simulink model "Cardiovascularmodel"  (Simulink 7.4)
settings: Solver=ode45  StartTime=0.0  StopTime=10.0  RelTol=1e-3
undefined symbols (not defined in the file): magnitude
(part 2 of 2)

== system Cardiovascularmodel/26 - 34/0.0.34i ==
  fsp : Inport  OutDataType=fixdt(1, 16)  OutScaling=2^0
  Constant : Constant  Value=0  OutDataType=fixdt(1, 16)  OutScaling=2^0
  Constant1 : Constant  OutDataType=fixdt(1, 16)  OutScaling=2^0
  D(V(u,ev)) : Constant  Value=5  OutDataType=fixdt(1, 16)  OutScaling=2^0
  G(V(e,sv)) : Constant  Value=-74.21  OutDataType=fixdt(1, 16)  OutScaling=2^0
  Math Function : Math  Operator=log  OutDataType=fixdt(1, 16)  OutScaling=2^0  SaturateOnIntegerOverflow=on
  Product : Product  OutDataType=fixdt(1, 16)  OutScaling=2^0  RndMeth=Zero
  Subtract1 : Sum  Inputs=++-  OutDataType=fixdt(1, 16)  OutScaling=2^-10
  Switch : Switch  Threshold=2.66  OutDataType=fixdt(1, 16)  OutScaling=2^0
  Variable Time Delay : VariableTransportDelay  MaximumDelay=10
  f(es,min) : Constant  Value=2.66  OutDataType=fixdt(1, 16)  OutScaling=2^0
  sigma(V(e,sv)) : Outport  OutDataType=fixdt(1, 16)  OutScaling=2^0
  wires:
  fsp/1 -> Switch/2, Variable Time Delay/1
  Switch/1 -> sigma(V(e,sv))/1
  Constant/1 -> Switch/3
  G(V(e,sv))/1 -> Product/1
  Product/1 -> Switch/1
  f(es,min)/1 -> Subtract1/3
  Variable Time Delay/1 -> Subtract1/2
  Constant1/1 -> Subtract1/1
  Subtract1/1 -> Math Function/1
  Math Function/1 -> Product/2
  D(V(u,ev))/1 -> Variable Time Delay/2

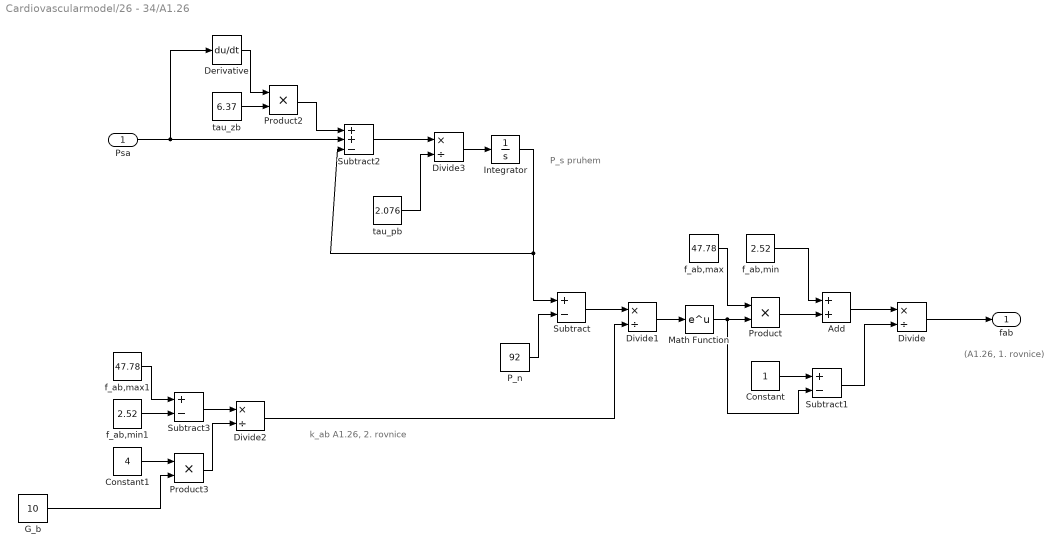
== system Cardiovascularmodel/26 - 34/A1.26 ==
  note: k_ab
      | A1.26, 2. rovnice
  note: P_s pruhem
  note: (A1.26, 1. rovnice)
  Psa : Inport  OutDataType=sfix(16)  OutScaling=2^0
  Add : Sum  OutDataType=sfix(16)  OutScaling=2^-10
  Constant : Constant  OutDataType=sfix(16)  OutScaling=2^0
  Constant1 : Constant  Value=4  OutDataType=sfix(16)  OutScaling=2^0
  Derivative : Derivative
  Divide : Product  Inputs=*/  OutDataType=sfix(16)  OutScaling=2^-10
  Divide1 : Product  Inputs=*/  OutDataType=sfix(16)  OutScaling=2^-10
  Divide2 : Product  Inputs=*/  OutDataType=sfix(16)  OutScaling=2^-10
  Divide3 : Product  Inputs=*/  OutDataType=fixdt(1, 16)  OutScaling=2^-10
  G_b : Constant  Value=10  OutDataType=sfix(16)  OutScaling=2^0
  Integrator : Integrator
  Math Function : Math  OutDataType=sfix(16)  OutScaling=2^0  SaturateOnIntegerOverflow=on
  P_n : Constant  Value=92  OutDataType=sfix(16)  OutScaling=2^0
  Product : Product  OutDataType=sfix(16)  OutScaling=2^0  RndMeth=Zero
  Product2 : Product  OutDataType=sfix(16)  OutScaling=2^0  RndMeth=Zero
  Product3 : Product  OutDataType=sfix(16)  OutScaling=2^0  RndMeth=Zero
  Subtract : Sum  Inputs=+-  OutDataType=sfix(16)  OutScaling=2^-10
  Subtract1 : Sum  Inputs=+-  OutDataType=sfix(16)  OutScaling=2^-10
  Subtract2 : Sum  Inputs=++-  OutDataType=sfix(16)  OutScaling=2^-10
  Subtract3 : Sum  Inputs=+-  OutDataType=sfix(16)  OutScaling=2^-10
  f_ab,max : Constant  Value=47.78  OutDataType=sfix(16)  OutScaling=2^0
  f_ab,max1 : Constant  Value=47.78  OutDataType=sfix(16)  OutScaling=2^0
  f_ab,min : Constant  Value=2.52  OutDataType=sfix(16)  OutScaling=2^0
  f_ab,min1 : Constant  Value=2.52  OutDataType=sfix(16)  OutScaling=2^0
  tau_pb : Constant  Value=2.076  OutDataType=sfix(16)  OutScaling=2^0
  tau_zb : Constant  Value=6.37  OutDataType=sfix(16)  OutScaling=2^0
  fab : Outport  OutDataType=sfix(16)  OutScaling=2^0
  wires:
  Divide/1 -> fab/1
  Add/1 -> Divide/1
  Product/1 -> Add/2
  f_ab,min/1 -> Add/1
  f_ab,max/1 -> Product/1
  Math Function/1 -> Product/2, Subtract1/2
  Divide1/1 -> Math Function/1
  Subtract/1 -> Divide1/1
  P_n/1 -> Subtract/2
  Subtract1/1 -> Divide/2
  Constant/1 -> Subtract1/1
  Psa/1 -> Subtract2/2, Derivative/1
  Product2/1 -> Subtract2/1
  tau_zb/1 -> Product2/2
  Divide2/1 -> Divide1/2
  Subtract3/1 -> Divide2/1
  f_ab,min1/1 -> Subtract3/2
  f_ab,max1/1 -> Subtract3/1
  Product3/1 -> Divide2/2
  Constant1/1 -> Product3/1
  G_b/1 -> Product3/2
  Derivative/1 -> Product2/1
  tau_pb/1 -> Divide3/2
  Subtract2/1 -> Divide3/1
  Divide3/1 -> Integrator/1
  Integrator/1 -> Subtract/1, Subtract2/3

== system Cardiovascularmodel/26 - 34/Elastance 0.0.32d ==
  delta Emax,lv : Inport  OutDataType=fixdt(1, 16)  OutScaling=2^0
  Emax,lv,0 : Constant  Value=2.392  OutDataType=fixdt(1, 16)  OutScaling=2^0
  Sum : Sum  Inputs=|++  OutDataType=fixdt(1, 16)  OutScaling=2^0
  E max,lv : Outport  OutDataType=fixdt(1, 16)  OutScaling=2^0
  wires:
  Sum/1 -> E max,lv/1
  Emax,lv,0/1 -> Sum/1
  delta Emax,lv/1 -> Sum/2

== system Cardiovascularmodel/26 - 34/Elastance dynamic 0.0.32b ==
  sigma (Emax,rv) : Inport  OutDataType=fixdt(1, 16)  OutScaling=2^0
  Constant : Constant  OutDataType=fixdt(1, 16)  OutScaling=2^0
  Constant1 : Constant  Value=-1  OutDataType=fixdt(1, 16)  OutScaling=2^0
  Divide : Product  Inputs=*/  OutDataType=fixdt(1, 16)  OutScaling=2^-10
  Integrator : Integrator
  Product : Product  OutDataType=fixdt(1, 16)  OutScaling=2^0  RndMeth=Zero
  Product1 : Product  OutDataType=fixdt(1, 16)  OutScaling=2^0  RndMeth=Zero
  Sum : Sum  Inputs=|++  OutDataType=fixdt(1, 16)  OutScaling=2^0
  tau(Emax,rv) : Constant  Value=8  OutDataType=fixdt(1, 16)  OutScaling=2^0
  delta  Emax,rv : Outport  OutDataType=fixdt(1, 16)  OutScaling=2^0
  wires:
  sigma (Emax,rv)/1 -> Sum/1
  Constant/1 -> Divide/1
  tau(Emax,rv)/1 -> Divide/2
  Divide/1 -> Product/1
  Constant1/1 -> Product1/2
  Product1/1 -> Sum/2
  Sum/1 -> Product/2
  Product/1 -> Integrator/1
  Integrator/1 -> delta  Emax,rv/1, Product1/1

== system Cardiovascularmodel/26 - 34/Elastance dynamic 0.0.32c ==
  delta Emax,rv : Inport  OutDataType=fixdt(1, 16)  OutScaling=2^0
  Emax,rv,0 : Constant  Value=1.412  OutDataType=fixdt(1, 16)  OutScaling=2^0
  Sum : Sum  Inputs=|++  OutDataType=fixdt(1, 16)  OutScaling=2^0
  E max,rv : Outport  OutDataType=fixdt(1, 16)  OutScaling=2^0
  wires:
  Sum/1 -> E max,rv/1
  Emax,rv,0/1 -> Sum/1
  delta Emax,rv/1 -> Sum/2

== system Cardiovascularmodel/26 - 34/Elastance dynamic 0.0.32e ==
  sigma (Emax,lv) : Inport  OutDataType=fixdt(1, 16)  OutScaling=2^0
  Constant : Constant  OutDataType=fixdt(1, 16)  OutScaling=2^0
  Constant1 : Constant  Value=-1  OutDataType=fixdt(1, 16)  OutScaling=2^0
  Divide : Product  Inputs=*/  OutDataType=fixdt(1, 16)  OutScaling=2^-10
  Integrator : Integrator
  Product : Product  OutDataType=fixdt(1, 16)  OutScaling=2^0  RndMeth=Zero
  Product1 : Product  OutDataType=fixdt(1, 16)  OutScaling=2^0  RndMeth=Zero
  Sum : Sum  Inputs=|++  OutDataType=fixdt(1, 16)  OutScaling=2^0
  tau(Emax,rv) : Constant  Value=8  OutDataType=fixdt(1, 16)  OutScaling=2^0
  delta  Emax,lv : Outport  OutDataType=fixdt(1, 16)  OutScaling=2^0
  wires:
  sigma (Emax,lv)/1 -> Sum/1
  Constant/1 -> Divide/1
  tau(Emax,rv)/1 -> Divide/2
  Divide/1 -> Product/1
  Constant1/1 -> Product1/2
  Product1/1 -> Sum/2
  Sum/1 -> Product/2
  Product/1 -> Integrator/1
  Integrator/1 -> delta  Emax,lv/1, Product1/1

== system Cardiovascularmodel/26 - 34/Heart rate dynamic 0.0.33a ==
  delta Ts(t) : Inport  OutDataType=fixdt(1, 16)  OutScaling=2^0
  delta Tv(t) : Inport  Port=2  OutDataType=fixdt(1, 16)  OutScaling=2^0
  Constant : Constant  Value=0.58  OutDataType=fixdt(1, 16)  OutScaling=2^0
  Sum : Sum  Inputs=|+++  OutDataType=fixdt(1, 16)  OutScaling=2^0
  T(t) : Outport  OutDataType=fixdt(1, 16)  OutScaling=2^0
  wires:
  delta Ts(t)/1 -> Sum/2
  Sum/1 -> T(t)/1
  delta Tv(t)/1 -> Sum/3
  Constant/1 -> Sum/1

== system Cardiovascularmodel/26 - 34/Heart rate dynamic 0.0.33b ==
  sigma (Ts) : Inport  OutDataType=fixdt(1, 16)  OutScaling=2^0
  Constant : Constant  OutDataType=fixdt(1, 16)  OutScaling=2^0
  Constant1 : Constant  Value=-1  OutDataType=fixdt(1, 16)  OutScaling=2^0
  Divide : Product  Inputs=*/  OutDataType=fixdt(1, 16)  OutScaling=2^-10
  Integrator : Integrator
  Product : Product  OutDataType=fixdt(1, 16)  OutScaling=2^0  RndMeth=Zero
  Product1 : Product  OutDataType=fixdt(1, 16)  OutScaling=2^0  RndMeth=Zero
  Sum : Sum  Inputs=|++  OutDataType=fixdt(1, 16)  OutScaling=2^0
  tau(Ts) : Constant  Value=2  OutDataType=fixdt(1, 16)  OutScaling=2^0
  delta Ts(t) : Outport  OutDataType=fixdt(1, 16)  OutScaling=2^0
  wires:
  sigma (Ts)/1 -> Sum/1
  Constant/1 -> Divide/1
  tau(Ts)/1 -> Divide/2
  Divide/1 -> Product/1
  Constant1/1 -> Product1/2
  Product1/1 -> Sum/2
  Sum/1 -> Product/2
  Product/1 -> Integrator/1
  Integrator/1 -> delta Ts(t)/1, Product1/1

== system Cardiovascularmodel/26 - 34/Heart rate dynamic 0.0.33c ==
  sigma (Tv) : Inport  OutDataType=fixdt(1, 16)  OutScaling=2^0
  Constant : Constant  OutDataType=fixdt(1, 16)  OutScaling=2^0
  Constant1 : Constant  Value=-1  OutDataType=fixdt(1, 16)  OutScaling=2^0
  Divide : Product  Inputs=*/  OutDataType=fixdt(1, 16)  OutScaling=2^-10
  Integrator : Integrator
  Product : Product  OutDataType=fixdt(1, 16)  OutScaling=2^0  RndMeth=Zero
  Product1 : Product  OutDataType=fixdt(1, 16)  OutScaling=2^0  RndMeth=Zero
  Sum : Sum  Inputs=|++  OutDataType=fixdt(1, 16)  OutScaling=2^0
  tau(Tv) : Constant  Value=1.5  OutDataType=fixdt(1, 16)  OutScaling=2^0
  delta Tv(t) : Outport  OutDataType=fixdt(1, 16)  OutScaling=2^0
  wires:
  sigma (Tv)/1 -> Sum/1
  Constant/1 -> Divide/1
  tau(Tv)/1 -> Divide/2
  Divide/1 -> Product/1
  Constant1/1 -> Product1/2
  Product1/1 -> Sum/2
  Sum/1 -> Product/2
  Product/1 -> Integrator/1
  Integrator/1 -> delta Tv(t)/1, Product1/1

== system Cardiovascularmodel/26 - 34/Peripheral Resistance Dynamic 0.0.31b ==
  Sigma (Rsp) : Inport  OutDataType=sfix(16)  OutScaling=2^0
  Add : Sum  Inputs=+-  OutDataType=sfix(16)  OutScaling=2^-10
  Constant : Constant  OutDataType=sfix(16)  OutScaling=2^0
  Divide : Product  Inputs=*/  OutDataType=sfix(16)  OutScaling=2^-10
  Product : Product  OutDataType=sfix(16)  OutScaling=2^0  RndMeth=Zero
  Rsp : Integrator
  tau (R,sp) : Constant  Value=6  OutDataType=sfix(16)  OutScaling=2^0
  d Delta R(sp) : Outport  OutDataType=sfix(16)  OutScaling=2^0
  wires:
  tau (R,sp)/1 -> Divide/2
  Constant/1 -> Divide/1
  Divide/1 -> Product/1
  Product/1 -> Rsp/1
  Rsp/1 -> d Delta R(sp)/1, Add/2
  Sigma (Rsp)/1 -> Add/1
  Add/1 -> Product/2

== system Cardiovascularmodel/26 - 34/Peripheral Resistance Dynamic 0.0.31e ==
  Sigma (Rmp) : Inport  OutDataType=sfix(16)  OutScaling=2^0
  Add : Sum  Inputs=+-  OutDataType=sfix(16)  OutScaling=2^-10
  Constant : Constant  OutDataType=sfix(16)  OutScaling=2^0
  Divide : Product  Inputs=*/  OutDataType=sfix(16)  OutScaling=2^-10
  Product : Product  OutDataType=sfix(16)  OutScaling=2^0  RndMeth=Zero
  Rsp : Integrator
  tau (R,mp) : Constant  Value=6  OutDataType=sfix(16)  OutScaling=2^0
  d Delta R(mp) : Outport  OutDataType=sfix(16)  OutScaling=2^0
  wires:
  tau (R,mp)/1 -> Divide/2
  Constant/1 -> Divide/1
  Divide/1 -> Product/1
  Product/1 -> Rsp/1
  Rsp/1 -> d Delta R(mp)/1, Add/2
  Sigma (Rmp)/1 -> Add/1
  Add/1 -> Product/2

== system Cardiovascularmodel/26 - 34/Peripheral Resistance Dynamic 0.0.31h ==
  Sigma (Rep) : Inport  OutDataType=sfix(16)  OutScaling=2^0
  Add : Sum  Inputs=+-  OutDataType=sfix(16)  OutScaling=2^-10
  Constant : Constant  OutDataType=sfix(16)  OutScaling=2^0
  Divide : Product  Inputs=*/  OutDataType=sfix(16)  OutScaling=2^-10
  Product : Product  OutDataType=sfix(16)  OutScaling=2^0  RndMeth=Zero
  Rsp : Integrator
  tau (R,mp) : Constant  Value=6  OutDataType=sfix(16)  OutScaling=2^0
  d Delta R(ep) : Outport  OutDataType=sfix(16)  OutScaling=2^0
  wires:
  tau (R,mp)/1 -> Divide/2
  Constant/1 -> Divide/1
  Divide/1 -> Product/1
  Product/1 -> Rsp/1
  Rsp/1 -> d Delta R(ep)/1, Add/2
  Sigma (Rep)/1 -> Add/1
  Add/1 -> Product/2

== system Cardiovascularmodel/26 - 34/Unstressed Volume 0.0.34a ==
  delta V u,mv : Inport  OutDataType=fixdt(1, 16)  OutScaling=2^0
  Sum : Sum  Inputs=|++  OutDataType=fixdt(1, 16)  OutScaling=2^0
  V(u,mv,0) : Constant  Value=503.26  OutDataType=fixdt(1, 16)  OutScaling=2^0
  V(u,mv) : Outport  OutDataType=fixdt(1, 16)  OutScaling=2^0
  wires:
  Sum/1 -> V(u,mv)/1
  V(u,mv,0)/1 -> Sum/1
  delta V u,mv/1 -> Sum/2

== system Cardiovascularmodel/26 - 34/Unstressed Volume 0.0.34b ==
  sigma (V u,mv) : Inport  OutDataType=fixdt(1, 16)  OutScaling=2^0
  Constant : Constant  OutDataType=fixdt(1, 16)  OutScaling=2^0
  Constant1 : Constant  Value=-1  OutDataType=fixdt(1, 16)  OutScaling=2^0
  Divide : Product  Inputs=*/  OutDataType=fixdt(1, 16)  OutScaling=2^-10
  Integrator : Integrator
  Product : Product  OutDataType=fixdt(1, 16)  OutScaling=2^0  RndMeth=Zero
  Product1 : Product  OutDataType=fixdt(1, 16)  OutScaling=2^0  RndMeth=Zero
  Sum : Sum  Inputs=|++  OutDataType=fixdt(1, 16)  OutScaling=2^0
  tau(V(u,mv)) : Constant  Value=20  OutDataType=fixdt(1, 16)  OutScaling=2^0
  delta  V(u,mv) : Outport  OutDataType=fixdt(1, 16)  OutScaling=2^0
  wires:
  sigma (V u,mv)/1 -> Sum/1
  Constant/1 -> Divide/1
  tau(V(u,mv))/1 -> Divide/2
  Divide/1 -> Product/1
  Constant1/1 -> Product1/2
  Product1/1 -> Sum/2
  Sum/1 -> Product/2
  Product/1 -> Integrator/1
  Integrator/1 -> delta  V(u,mv)/1, Product1/1

== system Cardiovascularmodel/26 - 34/Unstressed Volume 0.0.34d ==
  delta V u,sv : Inport  OutDataType=fixdt(1, 16)  OutScaling=2^0
  Sum : Sum  Inputs=|++  OutDataType=fixdt(1, 16)  OutScaling=2^0
  V(u,sv,0) : Constant  Value=1345.4  OutDataType=fixdt(1, 16)  OutScaling=2^0
  V(u,sv) : Outport  OutDataType=fixdt(1, 16)  OutScaling=2^0
  wires:
  Sum/1 -> V(u,sv)/1
  V(u,sv,0)/1 -> Sum/1
  delta V u,sv/1 -> Sum/2

== system Cardiovascularmodel/26 - 34/Unstressed Volume 0.0.34e ==
  sigma (V u,sv) : Inport  OutDataType=fixdt(1, 16)  OutScaling=2^0
  Constant : Constant  OutDataType=fixdt(1, 16)  OutScaling=2^0
  Constant1 : Constant  Value=-1  OutDataType=fixdt(1, 16)  OutScaling=2^0
  Divide : Product  Inputs=*/  OutDataType=fixdt(1, 16)  OutScaling=2^-10
  Integrator : Integrator
  Product : Product  OutDataType=fixdt(1, 16)  OutScaling=2^0  RndMeth=Zero
  Product1 : Product  OutDataType=fixdt(1, 16)  OutScaling=2^0  RndMeth=Zero
  Sum : Sum  Inputs=|++  OutDataType=fixdt(1, 16)  OutScaling=2^0
  tau(V(u,sv)) : Constant  Value=20  OutDataType=fixdt(1, 16)  OutScaling=2^0
  delta  V(u,sv) : Outport  OutDataType=fixdt(1, 16)  OutScaling=2^0
  wires:
  sigma (V u,sv)/1 -> Sum/1
  Constant/1 -> Divide/1
  tau(V(u,sv))/1 -> Divide/2
  Divide/1 -> Product/1
  Constant1/1 -> Product1/2
  Product1/1 -> Sum/2
  Sum/1 -> Product/2
  Product/1 -> Integrator/1
  Integrator/1 -> delta  V(u,sv)/1, Product1/1

== system Cardiovascularmodel/26 - 34/Unstressed Volume 0.0.34g ==
  delta V u,ev : Inport  OutDataType=fixdt(1, 16)  OutScaling=2^0
  Sum : Sum  Inputs=|++  OutDataType=fixdt(1, 16)  OutScaling=2^0
  V(u,ev,0) : Constant  Value=640.73  OutDataType=fixdt(1, 16)  OutScaling=2^0
  V(u,ev) : Outport  OutDataType=fixdt(1, 16)  OutScaling=2^0
  wires:
  Sum/1 -> V(u,ev)/1
  V(u,ev,0)/1 -> Sum/1
  delta V u,ev/1 -> Sum/2

== system Cardiovascularmodel/26 - 34/Unstressed Volume 0.0.34h ==
  sigma (V u,ev) : Inport  OutDataType=fixdt(1, 16)  OutScaling=2^0
  Constant : Constant  OutDataType=fixdt(1, 16)  OutScaling=2^0
  Constant1 : Constant  Value=-1  OutDataType=fixdt(1, 16)  OutScaling=2^0
  Divide : Product  Inputs=*/  OutDataType=fixdt(1, 16)  OutScaling=2^-10
  Integrator : Integrator
  Product : Product  OutDataType=fixdt(1, 16)  OutScaling=2^0  RndMeth=Zero
  Product1 : Product  OutDataType=fixdt(1, 16)  OutScaling=2^0  RndMeth=Zero
  Sum : Sum  Inputs=|++  OutDataType=fixdt(1, 16)  OutScaling=2^0
  tau(V(u,ev)) : Constant  Value=20  OutDataType=fixdt(1, 16)  OutScaling=2^0
  delta  V(u,ev) : Outport  OutDataType=fixdt(1, 16)  OutScaling=2^0
  wires:
  sigma (V u,ev)/1 -> Sum/1
  Constant/1 -> Divide/1
  tau(V(u,ev))/1 -> Divide/2
  Divide/1 -> Product/1
  Constant1/1 -> Product1/2
  Product1/1 -> Sum/2
  Sum/1 -> Product/2
  Product/1 -> Integrator/1
  Integrator/1 -> delta  V(u,ev)/1, Product1/1

== system Cardiovascularmodel/A1.19x/A1.19 ==
  T,sys : Inport  OutDataType=sfix(16)  OutScaling=2^0
  T(t) : Inport  Port=2  OutDataType=sfix(16)  OutScaling=2^0
  u(t) : Inport  Port=3  OutDataType=sfix(16)  OutScaling=2^0
  Constant : Constant  Value=0  OutDataType=sfix(16)  OutScaling=2^0
  Constant1 : Constant  Value=pi  OutDataType=sfix(16)  OutScaling=2^0
  Divide : Product  Inputs=/*  OutDataType=fixdt(1, 16)  OutScaling=2^-10
  Divide1 : Product  Inputs=*/  OutDataType=sfix(16)  OutScaling=2^-10
  Math Function : Math  Operator=magnitude^2  OutDataType=sfix(16)  OutScaling=2^0  SaturateOnIntegerOverflow=on
  Product : Product  OutDataType=sfix(16)  OutScaling=2^0  RndMeth=Zero
  Product1 : Product  OutDataType=sfix(16)  OutScaling=2^0  RndMeth=Zero
  Switch : Switch  Threshold=1/0.8333
  Trigonometric Function : Trigonometry
  fi(t) : Outport  OutDataType=sfix(16)  OutScaling=2^0
  wires:
  Switch/1 -> fi(t)/1
  T,sys/1 -> Divide1/2, Divide/1
  Constant/1 -> Switch/1
  Constant1/1 -> Product/1
  T(t)/1 -> Product/2
  Product/1 -> Divide1/1
  Divide1/1 -> Product1/2
  u(t)/1 -> Product1/1, Divide/2
  Product1/1 -> Trigonometric Function/1
  Trigonometric Function/1 -> Math Function/1
  Math Function/1 -> Switch/3
  Divide/1 -> Switch/2

== system Cardiovascularmodel/A1.19x/A1.19a ==
  ksi : Inport  OutDataType=sfix(16)  OutScaling=2^0
  Fcn : Fcn  Expr=abs(u - round(u))
  u(t) : Outport  OutDataType=sfix(16)  OutScaling=2^0
  wires:
  ksi/1 -> Fcn/1
  Fcn/1 -> u(t)/1

== system Cardiovascularmodel/A1.19x/A1.19b ==
  T(t) : Inport  OutDataType=sfix(16)  OutScaling=2^0
  Constant : Constant  OutDataType=sfix(16)  OutScaling=2^0
  Divide : Product  Inputs=*/  OutDataType=sfix(16)  OutScaling=2^-10
  Integrator : Integrator
  ksi : Outport  OutDataType=sfix(16)  OutScaling=2^0
  wires:
  Integrator/1 -> ksi/1
  Divide/1 -> Integrator/1
  T(t)/1 -> Divide/2
  Constant/1 -> Divide/1

== system Cardiovascularmodel/A1.19x/A1.19c ==
  Constant : Constant  OutDataType=sfix(16)  OutScaling=2^0
  Divide : Product  Inputs=*/  OutDataType=sfix(16)  OutScaling=2^-10
  Product : Product  OutDataType=sfix(16)  OutScaling=2^0  RndMeth=Zero
  Subtract : Sum  Inputs=+-  OutDataType=sfix(16)  OutScaling=2^-10
  T : Constant  Value=0.8333  OutDataType=sfix(16)  OutScaling=2^0
  T,sys0 : Constant  Value=0.5  OutDataType=sfix(16)  OutScaling=2^0
  ksys : Constant  Value=0.075  OutDataType=sfix(16)  OutScaling=2^0
  T,sys : Outport  OutDataType=sfix(16)  OutScaling=2^0
  wires:
  T,sys0/1 -> Subtract/1
  ksys/1 -> Product/1
  Divide/1 -> Product/2
  Constant/1 -> Divide/1
  T/1 -> Divide/2
  Product/1 -> Subtract/2
  Subtract/1 -> T,sys/1

== system Cardiovascularmodel/Left Ventricle 13-18, 35/0.0.35_Plv ==
  Pmax,lv : Inport  OutDataType=sfix(16)  OutScaling=2^0
  Rl,v : Inport  Port=2  OutDataType=sfix(16)  OutScaling=2^0
  Fo,l : Inport  Port=3  OutDataType=sfix(16)  OutScaling=2^0
  Product : Product  OutDataType=sfix(16)  OutScaling=2^0  RndMeth=Zero
  Subtract : Sum  Inputs=+-  OutDataType=sfix(16)  OutScaling=2^-10
  Plv : Outport  OutDataType=sfix(16)  OutScaling=2^0
  wires:
  Pmax,lv/1 -> Subtract/1
  Product/1 -> Subtract/2
  Rl,v/1 -> Product/1
  Fo,l/1 -> Product/2
  Subtract/1 -> Plv/1

== system Cardiovascularmodel/Left Ventricle 13-18, 35/A1.13 ==
  note: Pla
  Ppv : Inport  OutDataType=sfix(16)  OutScaling=2^0
  Fi,l : Inport  Port=2  OutDataType=sfix(16)  OutScaling=2^0
  Cla : Constant  Value=19.23  OutDataType=sfix(16)  OutScaling=2^0
  Constant : Constant  OutDataType=sfix(16)  OutScaling=2^0
  Divide : Product  Inputs=*/  OutDataType=sfix(16)  OutScaling=2^-10
  Divide1 : Product  Inputs=*/  OutDataType=sfix(16)  OutScaling=2^-10
  Integrator : Integrator
  Product : Product  OutDataType=sfix(16)  OutScaling=2^0  RndMeth=Zero
  Rpv : Constant  Value=0.0056  OutDataType=sfix(16)  OutScaling=2^0
  Subtract : Sum  Inputs=+-  OutDataType=sfix(16)  OutScaling=2^-10
  Subtract1 : Sum  Inputs=+-  OutDataType=sfix(16)  OutScaling=2^-10
  Pla : Outport  OutDataType=sfix(16)  OutScaling=2^0
  wires:
  Integrator/1 -> Pla/1, Subtract/2
  Constant/1 -> Divide/1
  Cla/1 -> Divide/2
  Ppv/1 -> Subtract/1
  Subtract/1 -> Divide1/1
  Rpv/1 -> Divide1/2
  Fi,l/1 -> Subtract1/2
  Divide1/1 -> Subtract1/1
  Subtract1/1 -> Product/2
  Divide/1 -> Product/1
  Product/1 -> Integrator/1

== system Cardiovascularmodel/Left Ventricle 13-18, 35/A1.14 ==
  Plv : Inport  OutDataType=sfix(16)  OutScaling=2^0
  Pla : Inport  Port=2  OutDataType=sfix(16)  OutScaling=2^0
  Constant : Constant  Value=0  OutDataType=sfix(16)  OutScaling=2^0
  Divide : Product  Inputs=*/  OutDataType=sfix(16)  OutScaling=2^-10
  Rla : Constant  Value=0.0025  OutDataType=sfix(16)  OutScaling=2^0
  Subtract : Sum  Inputs=+-  OutDataType=sfix(16)  OutScaling=2^-10
  Switch : Switch  Criteria=u2 > Threshold  OutDataType=sfix(16)  OutScaling=2^0
  Fi,l : Outport  OutDataType=sfix(16)  OutScaling=2^0
  wires:
  Rla/1 -> Divide/2
  Subtract/1 -> Divide/1, Switch/2
  Plv/1 -> Subtract/2
  Pla/1 -> Subtract/1
  Switch/1 -> Fi,l/1
  Divide/1 -> Switch/1
  Constant/1 -> Switch/3

== system Cardiovascularmodel/Left Ventricle 13-18, 35/A1.15 ==
  Fi,l : Inport  OutDataType=sfix(16)  OutScaling=2^0
  Fo,l : Inport  Port=2  OutDataType=sfix(16)  OutScaling=2^0
  Integrator : Integrator
  Subtract : Sum  Inputs=+-  OutDataType=sfix(16)  OutScaling=2^-10
  Vlv : Outport  OutDataType=sfix(16)  OutScaling=2^0
  wires:
  Integrator/1 -> Vlv/1
  Fi,l/1 -> Subtract/1
  Fo,l/1 -> Subtract/2
  Subtract/1 -> Integrator/1

== system Cardiovascularmodel/Left Ventricle 13-18, 35/A1.16 ==
  Psa : Inport  OutDataType=sfix(16)  OutScaling=2^0
  Pmax,lv : Inport  Port=2  OutDataType=sfix(16)  OutScaling=2^0
  Rlv : Inport  Port=3  OutDataType=sfix(16)  OutScaling=2^0
  Constant : Constant  Value=0  OutDataType=sfix(16)  OutScaling=2^0
  Divide : Product  Inputs=*/  OutDataType=sfix(16)  OutScaling=2^-10
  Subtract : Sum  Inputs=+-  OutDataType=sfix(16)  OutScaling=2^-10
  Switch : Switch  Criteria=u2 > Threshold  OutDataType=sfix(16)  OutScaling=2^0
  Fo,l : Outport  OutDataType=sfix(16)  OutScaling=2^0
  wires:
  Rlv/1 -> Divide/2
  Subtract/1 -> Divide/1, Switch/2
  Psa/1 -> Subtract/2
  Pmax,lv/1 -> Subtract/1
  Switch/1 -> Fo,l/1
  Constant/1 -> Switch/3
  Divide/1 -> Switch/1

== system Cardiovascularmodel/Left Ventricle 13-18, 35/A1.17 ==
  Pmax,lv : Inport  OutDataType=sfix(16)  OutScaling=2^0
  Product : Product  OutDataType=sfix(16)  OutScaling=2^0  RndMeth=Zero
  kR,lv : Constant  Value=3.75*10e-4  OutDataType=sfix(16)  OutScaling=2^0
  Rlv : Outport  OutDataType=sfix(16)  OutScaling=2^0
  wires:
  Pmax,lv/1 -> Product/2
  kR,lv/1 -> Product/1
  Product/1 -> Rlv/1

== system Cardiovascularmodel/Left Ventricle 13-18, 35/A1.18 ==
  fi(t) : Inport  OutDataType=sfix(16)  OutScaling=2^0
  Vlv : Inport  Port=2  OutDataType=sfix(16)  OutScaling=2^0
  Emax,lv : Inport  Port=3  OutDataType=sfix(16)  OutScaling=2^0
  Add : Sum  OutDataType=sfix(16)  OutScaling=2^-10
  Constant : Constant  OutDataType=sfix(16)  OutScaling=2^0
  Constant1 : Constant  OutDataType=sfix(16)  OutScaling=2^0
  Math Function : Math  OutDataType=sfix(16)  OutScaling=2^0  SaturateOnIntegerOverflow=on
  Po,lv : Constant  Value=1.5  OutDataType=sfix(16)  OutScaling=2^0
  Product : Product  Inputs=3  OutDataType=sfix(16)  OutScaling=2^0  RndMeth=Zero
  Product1 : Product  Inputs=3  OutDataType=sfix(16)  OutScaling=2^0  RndMeth=Zero
  Product2 : Product  OutDataType=sfix(16)  OutScaling=2^0  RndMeth=Zero
  Subtract : Sum  Inputs=+-  OutDataType=sfix(16)  OutScaling=2^-10
  Subtract1 : Sum  Inputs=+-  OutDataType=sfix(16)  OutScaling=2^-10
  Subtract2 : Sum  Inputs=+-  OutDataType=sfix(16)  OutScaling=2^-10
  "Vu,lv " : Constant  Value=16.77  OutDataType=sfix(16)  OutScaling=2^0
  kE,lv : Constant  Value=0.014  OutDataType=sfix(16)  OutScaling=2^0
  P,max,lv(t) : Outport  OutDataType=sfix(16)  OutScaling=2^0
  wires:
  fi(t)/1 -> Product/1, Subtract1/2
  Emax,lv/1 -> Product/2
  Subtract/1 -> Product/3
  Vlv/1 -> Subtract/1, Product2/2
  "Vu,lv "/1 -> Subtract/2
  Product/1 -> Add/1
  Product1/1 -> Add/2
  Subtract1/1 -> Product1/1
  Constant/1 -> Subtract1/1
  Po,lv/1 -> Product1/2
  Subtract2/1 -> Product1/3
  Math Function/1 -> Subtract2/1
  Product2/1 -> Math Function/1
  kE,lv/1 -> Product2/1
  Constant1/1 -> Subtract2/2
  Add/1 -> P,max,lv(t)/1

== system Cardiovascularmodel/Righ Ventricle 20-25,35/0.035_Prv ==
  Pmax,rv : Inport  OutDataType=sfix(16)  OutScaling=2^0
  Rr,v : Inport  Port=2  OutDataType=sfix(16)  OutScaling=2^0
  Fo,r : Inport  Port=3  OutDataType=sfix(16)  OutScaling=2^0
  Product : Product  OutDataType=sfix(16)  OutScaling=2^0  RndMeth=Zero
  Subtract : Sum  Inputs=+-  OutDataType=sfix(16)  OutScaling=2^-10
  Prv : Outport  OutDataType=sfix(16)  OutScaling=2^0
  wires:
  Pmax,rv/1 -> Subtract/1
  Product/1 -> Subtract/2
  Rr,v/1 -> Product/1
  Fo,r/1 -> Product/2
  Subtract/1 -> Prv/1

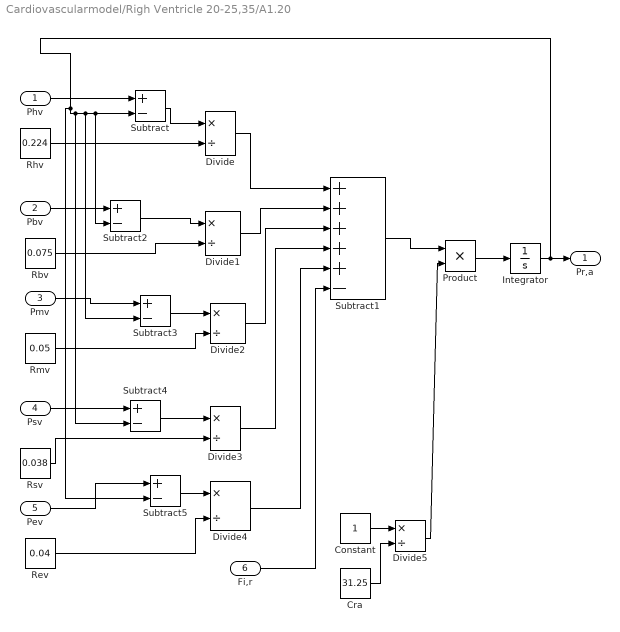
== system Cardiovascularmodel/Righ Ventricle 20-25,35/A1.20 ==
  Phv : Inport  OutDataType=sfix(16)  OutScaling=2^0
  Pbv : Inport  Port=2  OutDataType=sfix(16)  OutScaling=2^0
  Pmv : Inport  Port=3  OutDataType=sfix(16)  OutScaling=2^0
  Psv : Inport  Port=4  OutDataType=sfix(16)  OutScaling=2^0
  Pev : Inport  Port=5  OutDataType=sfix(16)  OutScaling=2^0
  Fi,r : Inport  Port=6  OutDataType=sfix(16)  OutScaling=2^0
  Constant : Constant  OutDataType=sfix(16)  OutScaling=2^0
  Cra : Constant  Value=31.25  OutDataType=sfix(16)  OutScaling=2^0
  Divide{,1..5} (6 alike) : Product  Inputs=*/  OutDataType=sfix(16)  OutScaling=2^-10
  Integrator : Integrator
  Product : Product  OutDataType=sfix(16)  OutScaling=2^0  RndMeth=Zero
  Rbv : Constant  Value=0.075  OutDataType=sfix(16)  OutScaling=2^0
  Rev : Constant  Value=0.04  OutDataType=sfix(16)  OutScaling=2^0
  Rhv : Constant  Value=0.224  OutDataType=sfix(16)  OutScaling=2^0
  Rmv : Constant  Value=0.05  OutDataType=sfix(16)  OutScaling=2^0
  Rsv : Constant  Value=0.038  OutDataType=sfix(16)  OutScaling=2^0
  Subtract{,2..5} (5 alike) : Sum  Inputs=+-  OutDataType=sfix(16)  OutScaling=2^-10
  Subtract1 : Sum  Inputs=+++++-  OutDataType=sfix(16)  OutScaling=2^-10
  Pr,a : Outport  OutDataType=sfix(16)  OutScaling=2^0
  wires:
  Integrator/1 -> Pr,a/1, Subtract/2, Subtract2/2, Subtract3/2, Subtract4/2, Subtract5/2
  Product/1 -> Integrator/1
  Subtract/1 -> Divide/1
  Phv/1 -> Subtract/1
  Rhv/1 -> Divide/2
  Divide/1 -> Subtract1/1
  Subtract2/1 -> Divide1/1
  Pbv/1 -> Subtract2/1
  Rbv/1 -> Divide1/2
  Divide1/1 -> Subtract1/2
  Divide2/1 -> Subtract1/3
  Subtract3/1 -> Divide2/1
  Pmv/1 -> Subtract3/1
  Rmv/1 -> Divide2/2
  Divide3/1 -> Subtract1/4
  Subtract4/1 -> Divide3/1
  Psv/1 -> Subtract4/1
  Rsv/1 -> Divide3/2
  Divide4/1 -> Subtract1/5
  Pev/1 -> Subtract5/1
  Subtract5/1 -> Divide4/1
  Rev/1 -> Divide4/2
  Subtract1/1 -> Product/1
  Fi,r/1 -> Subtract1/6
  Divide5/1 -> Product/2
  Constant/1 -> Divide5/1
  Cra/1 -> Divide5/2

== system Cardiovascularmodel/Righ Ventricle 20-25,35/A1.21 ==
  Pra : Inport  OutDataType=fixdt(1, 16)  OutScaling=2^0
  Prv : Inport  Port=2  OutDataType=sfix(16)  OutScaling=2^0
  Constant : Constant  Value=0  OutDataType=fixdt(1, 16)  OutScaling=2^0
  Divide : Product  Inputs=*/  OutDataType=fixdt(1, 16)  OutScaling=2^-10
  Rra : Constant  Value=0.0025  OutDataType=fixdt(1, 16)  OutScaling=2^0
  Subtract : Sum  Inputs=+-  OutDataType=fixdt(1, 16)  OutScaling=2^-10
  Switch : Switch  Criteria=u2 > Threshold  OutDataType=fixdt(1, 16)  OutScaling=2^0
  Fi,r : Outport  OutDataType=fixdt(1, 16)  OutScaling=2^0
  wires:
  Prv/1 -> Subtract/2
  Subtract/1 -> Divide/1, Switch/2
  Rra/1 -> Divide/2
  Switch/1 -> Fi,r/1
  Divide/1 -> Switch/1
  Constant/1 -> Switch/3
  Pra/1 -> Subtract/1

== system Cardiovascularmodel/Righ Ventricle 20-25,35/A1.22 ==
  Fi,r : Inport  OutDataType=fixdt(1, 16)  OutScaling=2^0
  Fo,r : Inport  Port=2  OutDataType=fixdt(1, 16)  OutScaling=2^0
  Integrator : Integrator
  Subtract : Sum  Inputs=+-  OutDataType=fixdt(1, 16)  OutScaling=2^-10
  Vrv : Outport  OutDataType=fixdt(1, 16)  OutScaling=2^0
  wires:
  Integrator/1 -> Vrv/1
  Fi,r/1 -> Subtract/1
  Fo,r/1 -> Subtract/2
  Subtract/1 -> Integrator/1

== system Cardiovascularmodel/Righ Ventricle 20-25,35/A1.23 ==
  Pmax,rv : Inport  OutDataType=fixdt(1, 16)  OutScaling=2^0
  Ppa : Inport  Port=2  OutDataType=fixdt(1, 16)  OutScaling=2^0
  Rrv : Inport  Port=3  OutDataType=sfix(16)  OutScaling=2^0
  Constant : Constant  Value=0  OutDataType=fixdt(1, 16)  OutScaling=2^0
  Divide : Product  Inputs=*/  OutDataType=fixdt(1, 16)  OutScaling=2^-10
  Subtract : Sum  Inputs=+-  OutDataType=fixdt(1, 16)  OutScaling=2^-10
  Switch : Switch  Criteria=u2 > Threshold  OutDataType=fixdt(1, 16)  OutScaling=2^0
  Fo,r : Outport  OutDataType=fixdt(1, 16)  OutScaling=2^0
  wires:
  Ppa/1 -> Subtract/2
  Pmax,rv/1 -> Subtract/1
  Subtract/1 -> Divide/1, Switch/2
  Rrv/1 -> Divide/2
  Switch/1 -> Fo,r/1
  Divide/1 -> Switch/1
  Constant/1 -> Switch/3

== system Cardiovascularmodel/Righ Ventricle 20-25,35/A1.24 ==
  Pmax,rv : Inport  OutDataType=sfix(16)  OutScaling=2^0
  Product : Product  OutDataType=sfix(16)  OutScaling=2^0  RndMeth=Zero
  kR,rv : Constant  Value=1.4*10e-3  OutDataType=sfix(16)  OutScaling=2^0
  Rrv : Outport  OutDataType=sfix(16)  OutScaling=2^0
  wires:
  Pmax,rv/1 -> Product/2
  kR,rv/1 -> Product/1
  Product/1 -> Rrv/1

== system Cardiovascularmodel/Righ Ventricle 20-25,35/A1.25 ==
  fi(t) : Inport  OutDataType=sfix(16)  OutScaling=2^0
  Vrv : Inport  Port=2  OutDataType=sfix(16)  OutScaling=2^0
  Emax.rv : Inport  Port=3  OutDataType=sfix(16)  OutScaling=2^0
  Constant : Constant  OutDataType=sfix(16)  OutScaling=2^0
  Constant1 : Constant  OutDataType=sfix(16)  OutScaling=2^0
  Math Function : Math  OutDataType=sfix(16)  OutScaling=2^0  SaturateOnIntegerOverflow=on
  Po,rv : Constant  Value=1.5  OutDataType=sfix(16)  OutScaling=2^0
  Product : Product  Inputs=3  OutDataType=sfix(16)  OutScaling=2^0  RndMeth=Zero
  Product1 : Product  Inputs=3  OutDataType=sfix(16)  OutScaling=2^0  RndMeth=Zero
  Product2 : Product  OutDataType=sfix(16)  OutScaling=2^0  RndMeth=Zero
  Subtract : Sum  Inputs=+-  OutDataType=sfix(16)  OutScaling=2^-10
  Subtract1 : Sum  Inputs=-+  OutDataType=sfix(16)  OutScaling=2^-10
  Subtract2 : Sum  Inputs=+-  OutDataType=sfix(16)  OutScaling=2^-10
  Sum : Sum  Inputs=|++  OutDataType=sfix(16)  OutScaling=2^0
  Vu,rv : Constant  Value=40.8  OutDataType=sfix(16)  OutScaling=2^0
  kErv : Constant  Value=0.11  OutDataType=sfix(16)  OutScaling=2^0
  Pmax,rv(t) : Outport  OutDataType=sfix(16)  OutScaling=2^0
  wires:
  fi(t)/1 -> Product/1, Subtract1/1
  Subtract/1 -> Product/2
  Vrv/1 -> Subtract/1, Product2/1
  Vu,rv/1 -> Subtract/2
  Emax.rv/1 -> Product/3
  Product/1 -> Sum/1
  Product1/1 -> Sum/2
  Subtract1/1 -> Product1/1
  Constant/1 -> Subtract1/2
  Po,rv/1 -> Product1/2
  Subtract2/1 -> Product1/3
  Math Function/1 -> Subtract2/1
  Product2/1 -> Math Function/1
  kErv/1 -> Product2/2
  Constant1/1 -> Subtract2/2
  Sum/1 -> Pmax,rv(t)/1
